simulink model "PRO_TestHarness"  (Simulink 8.6)
settings: Solver=ode45  StartTime=0.0  StopTime=10.0  RelTol=1e-3
PreLoadFcn:
  | addpath('./Workspace/')
  | load('./Workspace/EnvVar.mat')
  | if exist('tl_preloadfcn','file'), tl_preloadfcn(gcs,402); end
PostLoadFcn:
  | if exist('tl_postloadfcn','file'), tl_postloadfcn(gcs,402); end
InitFcn:
  | if exist('tlds_init','file'), tlds_init(gcs); end
StartFcn:
  | if exist('tlds_start','file'), tlds_start(gcs); end
StopFcn:
  | if exist('tlds_stop','file'), tlds_stop(gcs); end
undefined symbols (not defined in the file or in its folder): ddv, sigbuilder_block, Ts
libraries: tllib x19, simulink x2
(part 3 of 5)

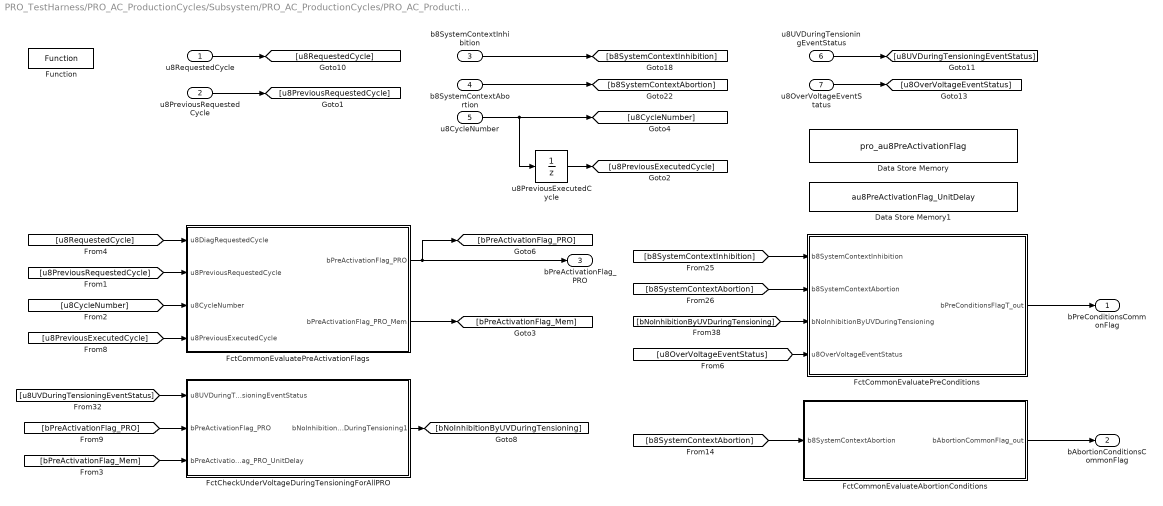
== system PRO_TestHarness/PRO_AC_ProductionCycles/Subsystem/PRO_AC_ProductionCycles/PRO_AC_ProductionCycles/PRO_runProductionCycles/PRO enabled/FctCommonPROManageInputs ==
  u8RequestedCycle : Inport  OutDataTypeStr=uint8  PortDimensions=1
  u8PreviousRequestedCycle : Inport  Port=2  OutDataTypeStr=uint8  PortDimensions=1
  b8SystemContextInhibition : Inport  Port=3  OutDataTypeStr=uint8  PortDimensions=1
  b8SystemContextAbortion : Inport  Port=4  OutDataTypeStr=uint8  PortDimensions=1
  u8CycleNumber : Inport  Port=5  PortDimensions=1
  u8UVDuringTensioningEventStatus : Inport  Port=6  OutDataTypeStr=uint8  PortDimensions=1
  u8OverVoltageEventStatus : Inport  Port=7
  Data Store Memory : DataStoreMemory  DataStoreName=pro_au8PreActivationFlag  ReadBeforeWriteMsg=warning  WriteAfterWriteMsg=warning  WriteAfterReadMsg=warning  InitialValue=ddv('PRO/pro_au8PreActivationFlag')  mask(TL_DataStoreMemory){data={'output',{'variable','PRO/pro_au8PreActivationFlag'},'autosar',{'softwarecomponent','AUTOLIV/SoftwareComponents/PRO/PRO_AC_ProductionCycles'},'date',736811.32661307871}}
      settings: CopyFcn=if exist('tl_reset_reviewflag') == 2, tl_reset_reviewflag(gcbh); end  DeleteFcn=if exist('delete_tlblock','file')==2,delete_tlblock(gcbh);end  NameChangeFcn=if exist('rename_tlblock','file')==2,rename_tlblock(gcbh);end  OpenFcn=if exist('tl_open_blockdlg','file')==2,tl_open_blockdlg(gcbh);else,open_system(gcbh,'parameter');end
      mask Help: eval(['if exist(''tl_online_help'',''file'') == 2, tl_online_help(''Topic'',''TL_DataStoreMemory''),else, web([''jar:file:///'',matlabroot,''/help/toolbox/simulink/help.jar!/slref/' lower(get_param(gcbh,'Blocktype')) '.html''], ''-helpbrowser''),end'])
      mask Display: plot([-0.05, 1.05, NaN, -0.05, 1.05],[.01, .01, NaN, .99, .99])
  Data Store Memory1 : DataStoreMemory  DataStoreName=au8PreActivationFlag_UnitDelay  ReadBeforeWriteMsg=warning  WriteAfterWriteMsg=warning  WriteAfterReadMsg=warning  InitialValue=ddv('PRO/pro_au8PreActivationFlag_UnitDelay')  mask(TL_DataStoreMemory){data={'output',{'variable','PRO/pro_au8PreActivationFlag_UnitDelay'},'autosar',{'softwarecomponent','AUTOLIV/SoftwareComponents/PRO/PRO_AC_ProductionCycles'},'date',736811.32661339117}}
      settings: CopyFcn=if exist('tl_reset_reviewflag') == 2, tl_reset_reviewflag(gcbh); end  DeleteFcn=if exist('delete_tlblock','file')==2,delete_tlblock(gcbh);end  NameChangeFcn=if exist('rename_tlblock','file')==2,rename_tlblock(gcbh);end  OpenFcn=if exist('tl_open_blockdlg','file')==2,tl_open_blockdlg(gcbh);else,open_system(gcbh,'parameter');end
      mask Help: eval(['if exist(''tl_online_help'',''file'') == 2, tl_online_help(''Topic'',''TL_DataStoreMemory''),else, web([''jar:file:///'',matlabroot,''/help/toolbox/simulink/help.jar!/slref/' lower(get_param(gcbh,'Blocktype')) '.html''], ''-helpbrowser''),end'])
      mask Display: plot([-0.05, 1.05, NaN, -0.05, 1.05],[.01, .01, NaN, .99, .99])
  FctCheckUnderVoltageDuringTensioningForAllPRO : Subsystem  TreatAsAtomicUnit=on
  FctCommonEvaluateAbortionConditions : Subsystem  TreatAsAtomicUnit=on
  FctCommonEvaluatePreActivationFlags : Subsystem  TreatAsAtomicUnit=on
  FctCommonEvaluatePreConditions : Subsystem  TreatAsAtomicUnit=on
  Function : tllib/Function  data={'stepfunctionname','ManageCommonInputsForAllPRO','stepfunctionclass','STATIC_FCN_ASR4','codecomment',['This function is in charge of' char(10) 'providing the following outputs:' char(10) '' char(10) '- the common PRO preconditions flag' char(10) '- the common PRO abortion flag' char(10) '- the consistent cycle number requested by diagnostic' char(10) '' char(10) 'according to the inputs:' char(10) '' char(10) '- the cycle requested by diagnostic' char(10) '- the complement of the cycle requested by diagnostic' char(10) '- inhibition context' char(10) '- abortion context'],'module','PRO_AC_ProductionCycles','date',736463.55388090282}  displayString=FUNCTION
  u8PreviousExecutedCycle : UnitDelay  InitialCondition=ddv('RTE_DEFINES/KU8_NO_CYCLE')  SampleTime=-1  mask(TL_UnitDelay){data={'output',{'name','$B','type','UInt8'},'state',{'name','X_$B','type','UInt8'},'date',736811.34423484956}}
      settings: CopyFcn=if exist('tl_reset_reviewflag') == 2, tl_reset_reviewflag(gcbh); end  DeleteFcn=if exist('delete_tlblock','file')==2,delete_tlblock(gcbh);end  NameChangeFcn=if exist('rename_tlblock','file')==2,rename_tlblock(gcbh);end  OpenFcn=if exist('tl_open_blockdlg','file')==2,tl_open_blockdlg(gcbh);else,open_system(gcbh,'parameter');end
      mask Help: eval(['if exist(''tl_online_help'',''file'') == 2, tl_online_help(''Topic'',''TL_UnitDelay''),else, web([''jar:file:///'',matlabroot,''/help/toolbox/simulink/help.jar!/slref/' lower(get_param(gcbh,'Blocktype')) '.html''], ''-helpbrowser''),end'])
      mask Display: plot([-0.05, 1.05, NaN, -0.05, 1.05],[.01, .01, NaN, .99, .99])
  bPreConditionsCommonFlag : Outport  InitialOutput=[0]
  bAbortionConditionsCommonFlag : Outport  Port=2  InitialOutput=[0]
  bPreActivationFlag_PRO : Outport  Port=3  InitialOutput=[0]
  wires:
  u8RequestedCycle/1 -> [u8RequestedCycle]
  FctCommonEvaluatePreConditions/1(bPreConditionsFlagT_out) -> bPreConditionsCommonFlag/1
  FctCommonEvaluateAbortionConditions/1(bAbortionCommonFlag_out) -> bAbortionConditionsCommonFlag/1
  b8SystemContextInhibition/1 -> [b8SystemContextInhibition]
  b8SystemContextAbortion/1 -> [b8SystemContextAbortion]
  [b8SystemContextAbortion] -> FctCommonEvaluatePreConditions/2(b8SystemContextAbortion)
  [b8SystemContextInhibition] -> FctCommonEvaluatePreConditions/1(b8SystemContextInhibition)
  [b8SystemContextAbortion] -> FctCommonEvaluateAbortionConditions/1(b8SystemContextAbortion)
  FctCommonEvaluatePreActivationFlags/1(bPreActivationFlag_PRO) -> [bPreActivationFlag_PRO], bPreActivationFlag_PRO/1
  [u8RequestedCycle] -> FctCommonEvaluatePreActivationFlags/1(u8DiagRequestedCycle)
  [u8PreviousRequestedCycle] -> FctCommonEvaluatePreActivationFlags/2(u8PreviousRequestedCycle)
  [u8CycleNumber] -> FctCommonEvaluatePreActivationFlags/3(u8CycleNumber)
  [u8PreviousExecutedCycle] -> FctCommonEvaluatePreActivationFlags/4(u8PreviousExecutedCycle)
  u8CycleNumber/1 -> u8PreviousExecutedCycle/1, [u8CycleNumber]
  u8PreviousExecutedCycle/1 -> [u8PreviousExecutedCycle]
  u8UVDuringTensioningEventStatus/1 -> [u8UVDuringTensioningEventStatus]
  FctCheckUnderVoltageDuringTensioningForAllPRO/1(bNoInhibitionByUVDuringTensioning1) -> [bNoInhibitionByUVDuringTensioning]
  [u8UVDuringTensioningEventStatus] -> FctCheckUnderVoltageDuringTensioningForAllPRO/1(u8UVDuringTensioningEventStatus)
  [bPreActivationFlag_PRO] -> FctCheckUnderVoltageDuringTensioningForAllPRO/2(bPreActivationFlag_PRO)
  [bNoInhibitionByUVDuringTensioning] -> FctCommonEvaluatePreConditions/3(bNoInhibitionByUVDuringTensioning)
  [u8OverVoltageEventStatus] -> FctCommonEvaluatePreConditions/4(u8OverVoltageEventStatus)
  u8OverVoltageEventStatus/1 -> [u8OverVoltageEventStatus]
  u8PreviousRequestedCycle/1 -> [u8PreviousRequestedCycle]
  [bPreActivationFlag_Mem] -> FctCheckUnderVoltageDuringTensioningForAllPRO/3(bPreActivationFlag_PRO_UnitDelay)
  FctCommonEvaluatePreActivationFlags/2(bPreActivationFlag_PRO_Mem) -> [bPreActivationFlag_Mem]

== system PRO_TestHarness/PRO_AC_ProductionCycles/Subsystem/PRO_AC_ProductionCycles/PRO_AC_ProductionCycles/PRO_runProductionCycles/PRO enabled/FctTrigAbortCycle_AllPRO ==
  u8ConsistentRequestedCycle : Inport  OutDataTypeStr=uint8  PortDimensions=1
  u8PreviousConsistentRequestedCycle1 : Inport  Port=2  OutDataTypeStr=uint8  PortDimensions=1
  u8ExecutedCycle : Inport  Port=3  PortDimensions=1
  bPreConditionsCommonFlag : Inport  Port=4
  bAbortionCommonFlag : Inport  Port=5  PortDimensions=1
  bPreActivation_PRO : Inport  Port=6
  Constant : Constant  Value=ddv('PRO/KU8_NB_PROD_CYCLE')  mask(TL_Constant){data={'output',{'variable','PRO/KU8_NB_PROD_CYCLE'},'date',736169.6247268056}}
      settings: CopyFcn=if exist('tl_reset_reviewflag') == 2, tl_reset_reviewflag(gcbh); end  DeleteFcn=if exist('delete_tlblock','file')==2,delete_tlblock(gcbh);end  NameChangeFcn=if exist('rename_tlblock','file')==2,rename_tlblock(gcbh);end  OpenFcn=if exist('tl_open_blockdlg','file')==2,tl_open_blockdlg(gcbh);else,open_system(gcbh,'parameter');end
      mask Help: eval(['if exist(''tl_online_help'',''file'') == 2, tl_online_help(''Topic'',''TL_Constant''),else, web([''jar:file:///'',matlabroot,''/help/toolbox/simulink/help.jar!/slref/' lower(get_param(gcbh,'Blocktype')) '.html''], ''-helpbrowser''),end'])
      mask Display: plot([-0.05, 1.05, NaN, -0.05, 1.05],[.01, .01, NaN, .99, .99])
  For Iterator Subsystem : Subsystem  TreatAsAtomicUnit=on
  Function : tllib/Function  data={'stepfunctionname','DecideForAllPRO','stepfunctionclass','STATIC_FCN_ASR4','codecomment',['This function is in charge of' char(10) 'providing the following outputs:' char(10) '' char(10) '- Trigger flags for PRO1 and PRO2 cycles' char(10) '- Pre Activation flags for PRO1 and PRO2 cycles' char(10) '- Pre Conditions flags for PRO1 and PRO2 cycles' char(10) '- Triggering Sources for PRO1 and PRO2 cycles' char(10) '' char(10) 'according to the inputs:' char(10) '' char(10) '- executed cycle number' char(10) '- consistent current cycle requested by diagnostic' char(10) '- common PRO preconditions flag' char(10) '- common PRO abortion flag'],'module','PRO_AC_ProductionCycles','date',736463.55393209495}  displayString=FUNCTION
  s8TempIndex : DataTypeConversion  mask(TL_Rescaler){data={'output',{'name','$B','type','Int8'},'date',736169.64125245367}}
      settings: DeleteFcn=if exist('delete_tlblock','file')==2,delete_tlblock(gcbh);end  NameChangeFcn=if exist('rename_tlblock','file')==2,rename_tlblock(gcbh);end  OpenFcn=if exist('tl_open_blockdlg','file')==2,tl_open_blockdlg(gcbh);else,open_system(gcbh,'parameter');end
      mask Help: eval(['if exist(''tl_online_help'',''file'') == 2, tl_online_help(''Topic'',''TL_Rescaler''),else, web([''jar:file:///'',matlabroot,''/help/toolbox/simulink/help.jar!/slref/' lower(get_param(gcbh,'Blocktype')) '.html''], ''-helpbrowser''),end'])
      mask Display: plot([-0.05, 1.05, NaN, -0.05, 1.05],[.01, .01, NaN, .99, .99])
  psrAlgoFlags_PRO1 : Outport
  psrAlgoFlags_PRO2 : Outport  Port=2
  wires:
  u8ExecutedCycle/1 -> [u8ExecutedCycle]
  bAbortionCommonFlag/1 -> [bAbortionCommonFlag]
  bPreConditionsCommonFlag/1 -> [bPreConditionsCommonFlag]
  u8ConsistentRequestedCycle/1 -> [u8RequestedCycle]
  bPreActivation_PRO/1 -> [bPreActivation_PRO]
  u8PreviousConsistentRequestedCycle1/1 -> [u8PreviousRequestedCycle]
  Constant/1 -> s8TempIndex/1
  s8TempIndex/1 -> For Iterator Subsystem/1(Iteration Limit)
  [bPreConditionsCommonFlag] -> For Iterator Subsystem/5(bPreConditionsCommonFlag)
  [bPreActivation_PRO] -> For Iterator Subsystem/7(bPreActivation_PRO)
  [bAbortionCommonFlag] -> For Iterator Subsystem/6(bAbortionCommonFlag)
  [u8PreviousRequestedCycle] -> For Iterator Subsystem/3(u8PreviousConsistentRequestedCycle1)
  [u8RequestedCycle] -> For Iterator Subsystem/2(u8ConsistentRequestedCycle)
  [u8ExecutedCycle] -> For Iterator Subsystem/4(u8ExecutedCycle)
  For Iterator Subsystem/1(psrAlgoFlags_PRO1) -> psrAlgoFlags_PRO1/1
  For Iterator Subsystem/2(psrAlgoFlags_PRO2) -> psrAlgoFlags_PRO2/1

== system PRO_TestHarness/PRO_AC_ProductionCycles/Subsystem/PRO_AC_ProductionCycles/PRO_AC_ProductionCycles/PRO_runProductionCycles/SCA_runCheckSystemContext1/If Action Subsystem1 ==
  Action Port : ActionPort  ActionType=then
  Data Store Read1 : DataStoreRead  DataStoreName=b8CyclesInhibitedByDTC  mask(TL_DataStoreRead){data={'date',735893.56911439809}}
      settings: DeleteFcn=if exist('delete_tlblock','file')==2,delete_tlblock(gcbh);end  NameChangeFcn=if exist('rename_tlblock','file')==2,rename_tlblock(gcbh);end  OpenFcn=if exist('tl_open_blockdlg','file')==2,tl_open_blockdlg(gcbh);else,open_system(gcbh,'parameter');end
      mask Help: eval(['if exist(''tl_online_help'',''file'') == 2, tl_online_help(''Topic'',''TL_DataStoreRead''),else, web([''jar:file:///'',matlabroot,''/help/toolbox/simulink/help.jar!/slref/' lower(get_param(gcbh,'Blocktype')) '.html''], ''-helpbrowser''),end'])
      mask Display: plot([-0.05, 1.05, NaN, -0.05, 1.05],[.01, .01, NaN, .99, .99])
  Out1 : Outport
  wires:
  Data Store Read1/1 -> Out1/1

== system PRO_TestHarness/PRO_AC_ProductionCycles/Subsystem/PRO_AC_ProductionCycles/PRO_AC_ProductionCycles/PRO_runProductionCycles/SCA_runCheckSystemContext1/If Action Subsystem2 ==
  Action Port : ActionPort  ActionType=else
  Data Store Read2 : DataStoreRead  DataStoreName=b8CyclesAbortedByDTC  mask(TL_DataStoreRead){data={'date',735893.56919435191}}
      settings: DeleteFcn=if exist('delete_tlblock','file')==2,delete_tlblock(gcbh);end  NameChangeFcn=if exist('rename_tlblock','file')==2,rename_tlblock(gcbh);end  OpenFcn=if exist('tl_open_blockdlg','file')==2,tl_open_blockdlg(gcbh);else,open_system(gcbh,'parameter');end
      mask Help: eval(['if exist(''tl_online_help'',''file'') == 2, tl_online_help(''Topic'',''TL_DataStoreRead''),else, web([''jar:file:///'',matlabroot,''/help/toolbox/simulink/help.jar!/slref/' lower(get_param(gcbh,'Blocktype')) '.html''], ''-helpbrowser''),end'])
      mask Display: plot([-0.05, 1.05, NaN, -0.05, 1.05],[.01, .01, NaN, .99, .99])
  Out1 : Outport
  wires:
  Data Store Read2/1 -> Out1/1

== system PRO_TestHarness/PRO_AC_ProductionCycles/Subsystem/PRO_AC_ProductionCycles/PRO_AC_ProductionCycles/PRO_runProductionCycles/SCA_runCheckSystemContext2/If Action Subsystem1 ==
  Action Port : ActionPort  ActionType=then
  Data Store Read1 : DataStoreRead  DataStoreName=b8CyclesInhibitedByDTC  mask(TL_DataStoreRead){data={'date',735893.5693029745}}
      settings: DeleteFcn=if exist('delete_tlblock','file')==2,delete_tlblock(gcbh);end  NameChangeFcn=if exist('rename_tlblock','file')==2,rename_tlblock(gcbh);end  OpenFcn=if exist('tl_open_blockdlg','file')==2,tl_open_blockdlg(gcbh);else,open_system(gcbh,'parameter');end
      mask Help: eval(['if exist(''tl_online_help'',''file'') == 2, tl_online_help(''Topic'',''TL_DataStoreRead''),else, web([''jar:file:///'',matlabroot,''/help/toolbox/simulink/help.jar!/slref/' lower(get_param(gcbh,'Blocktype')) '.html''], ''-helpbrowser''),end'])
      mask Display: plot([-0.05, 1.05, NaN, -0.05, 1.05],[.01, .01, NaN, .99, .99])
  Out1 : Outport
  wires:
  Data Store Read1/1 -> Out1/1

== system PRO_TestHarness/PRO_AC_ProductionCycles/Subsystem/PRO_AC_ProductionCycles/PRO_AC_ProductionCycles/PRO_runProductionCycles/SCA_runCheckSystemContext2/If Action Subsystem2 ==
  Action Port : ActionPort  ActionType=else
  Data Store Read2 : DataStoreRead  DataStoreName=b8CyclesAbortedByDTC  mask(TL_DataStoreRead){data={'date',735893.56938277779}}
      settings: DeleteFcn=if exist('delete_tlblock','file')==2,delete_tlblock(gcbh);end  NameChangeFcn=if exist('rename_tlblock','file')==2,rename_tlblock(gcbh);end  OpenFcn=if exist('tl_open_blockdlg','file')==2,tl_open_blockdlg(gcbh);else,open_system(gcbh,'parameter');end
      mask Help: eval(['if exist(''tl_online_help'',''file'') == 2, tl_online_help(''Topic'',''TL_DataStoreRead''),else, web([''jar:file:///'',matlabroot,''/help/toolbox/simulink/help.jar!/slref/' lower(get_param(gcbh,'Blocktype')) '.html''], ''-helpbrowser''),end'])
      mask Display: plot([-0.05, 1.05, NaN, -0.05, 1.05],[.01, .01, NaN, .99, .99])
  Out1 : Outport
  wires:
  Data Store Read2/1 -> Out1/1

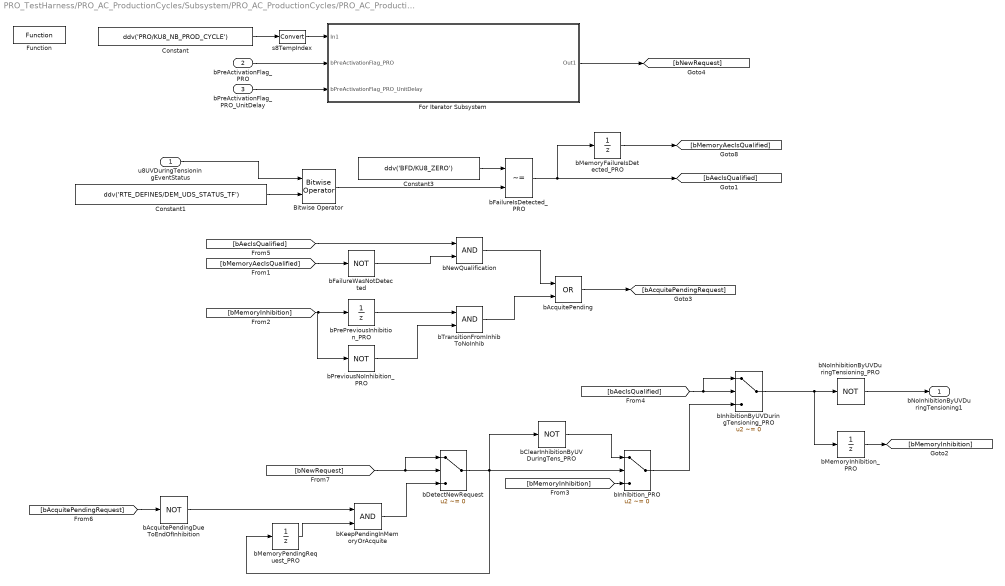
== system PRO_TestHarness/PRO_AC_ProductionCycles/Subsystem/PRO_AC_ProductionCycles/PRO_AC_ProductionCycles/PRO_runProductionCycles/PRO enabled/FctCommonPROManageInputs/FctCheckUnderVoltageDuringTensioningForAllPRO ==
  u8UVDuringTensioningEventStatus : Inport  OutDataTypeStr=uint8  PortDimensions=1
  bPreActivationFlag_PRO : Inport  Port=2
  bPreActivationFlag_PRO_UnitDelay : Inport  Port=3
  Bitwise Operator : tllib/Bitwise Operator  logicop=AND  UseBitMask=off  NumInputPorts=2  BitMask=bin2dec('11011001')  BitMaskRealWorld=Stored Integer  data={'date',736229.48596016201}
  Constant : Constant  Value=ddv('PRO/KU8_NB_PROD_CYCLE')  mask(TL_Constant){data={'output',{'variable','PRO/KU8_NB_PROD_CYCLE'},'date',736169.6247268056}}
      settings: CopyFcn=if exist('tl_reset_reviewflag') == 2, tl_reset_reviewflag(gcbh); end  DeleteFcn=if exist('delete_tlblock','file')==2,delete_tlblock(gcbh);end  NameChangeFcn=if exist('rename_tlblock','file')==2,rename_tlblock(gcbh);end  OpenFcn=if exist('tl_open_blockdlg','file')==2,tl_open_blockdlg(gcbh);else,open_system(gcbh,'parameter');end
      mask Help: eval(['if exist(''tl_online_help'',''file'') == 2, tl_online_help(''Topic'',''TL_Constant''),else, web([''jar:file:///'',matlabroot,''/help/toolbox/simulink/help.jar!/slref/' lower(get_param(gcbh,'Blocktype')) '.html''], ''-helpbrowser''),end'])
      mask Display: plot([-0.05, 1.05, NaN, -0.05, 1.05],[.01, .01, NaN, .99, .99])
  Constant1 : Constant  Value=ddv('RTE_DEFINES/DEM_UDS_STATUS_TF')  OutDataTypeStr=uint8  mask(TL_Constant){data={'output',{'variable','RTE_DEFINES/DEM_UDS_STATUS_TF'},'date',736811.33641298616}}
      settings: DeleteFcn=if exist('delete_tlblock','file')==2,delete_tlblock(gcbh);end  NameChangeFcn=if exist('rename_tlblock','file')==2,rename_tlblock(gcbh);end  OpenFcn=if exist('tl_open_blockdlg','file')==2,tl_open_blockdlg(gcbh);else,open_system(gcbh,'parameter');end
      mask Help: eval(['if exist(''tl_online_help'',''file'') == 2, tl_online_help(''Topic'',''TL_Constant''),else, web([''jar:file:///'',matlabroot,''/help/toolbox/simulink/help.jar!/slref/' lower(get_param(gcbh,'Blocktype')) '.html''], ''-helpbrowser''),end'])
      mask Display: plot([-0.05, 1.05, NaN, -0.05, 1.05],[.01, .01, NaN, .99, .99])
  Constant3 : Constant  Value=ddv('BFD/KU8_ZERO')  OutDataTypeStr=uint8  mask(TL_Constant){data={'output',{'variable','BFD/KU8_ZERO'},'date',736229.48516401625}}
      settings: DeleteFcn=if exist('delete_tlblock','file')==2,delete_tlblock(gcbh);end  NameChangeFcn=if exist('rename_tlblock','file')==2,rename_tlblock(gcbh);end  OpenFcn=if exist('tl_open_blockdlg','file')==2,tl_open_blockdlg(gcbh);else,open_system(gcbh,'parameter');end
      mask Help: eval(['if exist(''tl_online_help'',''file'') == 2, tl_online_help(''Topic'',''TL_Constant''),else, web([''jar:file:///'',matlabroot,''/help/toolbox/simulink/help.jar!/slref/' lower(get_param(gcbh,'Blocktype')) '.html''], ''-helpbrowser''),end'])
      mask Display: plot([-0.05, 1.05, NaN, -0.05, 1.05],[.01, .01, NaN, .99, .99])
  For Iterator Subsystem : Subsystem  TreatAsAtomicUnit=on
  Function : tllib/Function  data={'stepfunctionname','ExecuteBP_CheckUnderVoltageDuringTensioningForAllPRO','stepfunctionclass','STATIC_FCN_ASR4','codecomment',['This function is in charge of' char(10) 'providing the following outputs:' char(10) '' char(10) '- detection of temperature in correct range' char(10) '' char(10) 'according to the inputs:' char(10) '' char(10) '- the filtered internal temperature'],'module','PRO_AC_ProductionCycles','date',736463.55388949078}  displayString=FUNCTION
  bAcquitePending : Logic  Operator=OR  AllPortsSameDT=off  OutDataTypeStr=boolean  mask(TL_LogicalOperator){data={'output',{'name','$B'},'date',735916.64078504627}}
      settings: DeleteFcn=if exist('delete_tlblock','file')==2,delete_tlblock(gcbh);end  NameChangeFcn=if exist('rename_tlblock','file')==2,rename_tlblock(gcbh);end  OpenFcn=if exist('tl_open_blockdlg','file')==2,tl_open_blockdlg(gcbh);else,open_system(gcbh,'parameter');end
      mask Help: eval(['if exist(''tl_online_help'',''file'') == 2, tl_online_help(''Topic'',''TL_LogicalOperator''),else, web([''jar:file:///'',matlabroot,''/help/toolbox/simulink/help.jar!/slref/' lower(get_param(gcbh,'Blocktype')) '.html''], ''-helpbrowser''),end'])
      mask Display: plot([-0.05, 1.05, NaN, -0.05, 1.05],[.01, .01, NaN, .99, .99])
  bAcquitePendingDueToEndOfInhibition : Logic  Operator=NOT  Inputs=1  AllPortsSameDT=off  OutDataTypeStr=boolean  mask(TL_LogicalOperator){data={'output',{'name','$B'},'date',735910.63061995374}}
      settings: DeleteFcn=if exist('delete_tlblock','file')==2,delete_tlblock(gcbh);end  NameChangeFcn=if exist('rename_tlblock','file')==2,rename_tlblock(gcbh);end  OpenFcn=if exist('tl_open_blockdlg','file')==2,tl_open_blockdlg(gcbh);else,open_system(gcbh,'parameter');end
      mask Help: eval(['if exist(''tl_online_help'',''file'') == 2, tl_online_help(''Topic'',''TL_LogicalOperator''),else, web([''jar:file:///'',matlabroot,''/help/toolbox/simulink/help.jar!/slref/' lower(get_param(gcbh,'Blocktype')) '.html''], ''-helpbrowser''),end'])
      mask Display: plot([-0.05, 1.05, NaN, -0.05, 1.05],[.01, .01, NaN, .99, .99])
  bClearInhibitionByUVDuringTens_PRO : Logic  Operator=NOT  Inputs=1  AllPortsSameDT=off  OutDataTypeStr=boolean  mask(TL_LogicalOperator){data={'output',{'name','$B'},'date',735910.63061995374}}
      settings: DeleteFcn=if exist('delete_tlblock','file')==2,delete_tlblock(gcbh);end  NameChangeFcn=if exist('rename_tlblock','file')==2,rename_tlblock(gcbh);end  OpenFcn=if exist('tl_open_blockdlg','file')==2,tl_open_blockdlg(gcbh);else,open_system(gcbh,'parameter');end
      mask Help: eval(['if exist(''tl_online_help'',''file'') == 2, tl_online_help(''Topic'',''TL_LogicalOperator''),else, web([''jar:file:///'',matlabroot,''/help/toolbox/simulink/help.jar!/slref/' lower(get_param(gcbh,'Blocktype')) '.html''], ''-helpbrowser''),end'])
      mask Display: plot([-0.05, 1.05, NaN, -0.05, 1.05],[.01, .01, NaN, .99, .99])
  bDetectNewRequest : Switch  Criteria=u2 ~= 0  mask(TL_Switch){data={'output',{'name','$B','type','Bool'},'date',735907.68205655087}}
      settings: CopyFcn=if exist('tl_reset_reviewflag') == 2, tl_reset_reviewflag(gcbh); end  DeleteFcn=if exist('delete_tlblock','file')==2,delete_tlblock(gcbh);end  NameChangeFcn=if exist('rename_tlblock','file')==2,rename_tlblock(gcbh);end  OpenFcn=if exist('tl_open_blockdlg','file')==2,tl_open_blockdlg(gcbh);else,open_system(gcbh,'parameter');end
      mask Help: eval(['if exist(''tl_online_help'',''file'') == 2, tl_online_help(''Topic'',''TL_Switch''),else, web([''jar:file:///'',matlabroot,''/help/toolbox/simulink/help.jar!/slref/' lower(get_param(gcbh,'Blocktype')) '.html''], ''-helpbrowser''),end'])
      mask Display: plot([-0.05, 1.05, NaN, -0.05, 1.05],[.01, .01, NaN, .99, .99])
  bFailureIsDetected_PRO : RelationalOperator  Operator=~=  OutDataTypeStr=boolean  mask(TL_RelationalOperator){data={'output',{'name','$B'},'date',736229.48553751153}}
      settings: DeleteFcn=if exist('delete_tlblock','file')==2,delete_tlblock(gcbh);end  NameChangeFcn=if exist('rename_tlblock','file')==2,rename_tlblock(gcbh);end  OpenFcn=if exist('tl_open_blockdlg','file')==2,tl_open_blockdlg(gcbh);else,open_system(gcbh,'parameter');end
      mask Help: eval(['if exist(''tl_online_help'',''file'') == 2, tl_online_help(''Topic'',''TL_RelationalOperator''),else, web([''jar:file:///'',matlabroot,''/help/toolbox/simulink/help.jar!/slref/' lower(get_param(gcbh,'Blocktype')) '.html''], ''-helpbrowser''),end'])
      mask Display: plot([-0.05, 1.05, NaN, -0.05, 1.05],[.01, .01, NaN, .99, .99])
  bFailureWasNotDetected : Logic  Operator=NOT  Inputs=1  AllPortsSameDT=off  OutDataTypeStr=boolean  mask(TL_LogicalOperator){data={'output',{'name','$B'},'date',735910.63061995374}}
      settings: DeleteFcn=if exist('delete_tlblock','file')==2,delete_tlblock(gcbh);end  NameChangeFcn=if exist('rename_tlblock','file')==2,rename_tlblock(gcbh);end  OpenFcn=if exist('tl_open_blockdlg','file')==2,tl_open_blockdlg(gcbh);else,open_system(gcbh,'parameter');end
      mask Help: eval(['if exist(''tl_online_help'',''file'') == 2, tl_online_help(''Topic'',''TL_LogicalOperator''),else, web([''jar:file:///'',matlabroot,''/help/toolbox/simulink/help.jar!/slref/' lower(get_param(gcbh,'Blocktype')) '.html''], ''-helpbrowser''),end'])
      mask Display: plot([-0.05, 1.05, NaN, -0.05, 1.05],[.01, .01, NaN, .99, .99])
  bInhibitionByUVDuringTensioning_PRO : Switch  Criteria=u2 ~= 0  mask(TL_Switch){data={'output',{'name','$B','type','Bool'},'date',735907.68205655087}}
      settings: CopyFcn=if exist('tl_reset_reviewflag') == 2, tl_reset_reviewflag(gcbh); end  DeleteFcn=if exist('delete_tlblock','file')==2,delete_tlblock(gcbh);end  NameChangeFcn=if exist('rename_tlblock','file')==2,rename_tlblock(gcbh);end  OpenFcn=if exist('tl_open_blockdlg','file')==2,tl_open_blockdlg(gcbh);else,open_system(gcbh,'parameter');end
      mask Help: eval(['if exist(''tl_online_help'',''file'') == 2, tl_online_help(''Topic'',''TL_Switch''),else, web([''jar:file:///'',matlabroot,''/help/toolbox/simulink/help.jar!/slref/' lower(get_param(gcbh,'Blocktype')) '.html''], ''-helpbrowser''),end'])
      mask Display: plot([-0.05, 1.05, NaN, -0.05, 1.05],[.01, .01, NaN, .99, .99])
  bInhibition_PRO : Switch  Criteria=u2 ~= 0  mask(TL_Switch){data={'output',{'name','$B','type','Bool'},'date',735907.68205655087}}
      settings: CopyFcn=if exist('tl_reset_reviewflag') == 2, tl_reset_reviewflag(gcbh); end  DeleteFcn=if exist('delete_tlblock','file')==2,delete_tlblock(gcbh);end  NameChangeFcn=if exist('rename_tlblock','file')==2,rename_tlblock(gcbh);end  OpenFcn=if exist('tl_open_blockdlg','file')==2,tl_open_blockdlg(gcbh);else,open_system(gcbh,'parameter');end
      mask Help: eval(['if exist(''tl_online_help'',''file'') == 2, tl_online_help(''Topic'',''TL_Switch''),else, web([''jar:file:///'',matlabroot,''/help/toolbox/simulink/help.jar!/slref/' lower(get_param(gcbh,'Blocktype')) '.html''], ''-helpbrowser''),end'])
      mask Display: plot([-0.05, 1.05, NaN, -0.05, 1.05],[.01, .01, NaN, .99, .99])
  bKeepPendingInMemoryOrAcquite : Logic  AllPortsSameDT=off  OutDataTypeStr=boolean  mask(TL_LogicalOperator){data={'output',{'name','$B'},'date',735907.68610908568}}
      settings: DeleteFcn=if exist('delete_tlblock','file')==2,delete_tlblock(gcbh);end  NameChangeFcn=if exist('rename_tlblock','file')==2,rename_tlblock(gcbh);end  OpenFcn=if exist('tl_open_blockdlg','file')==2,tl_open_blockdlg(gcbh);else,open_system(gcbh,'parameter');end
      mask Help: eval(['if exist(''tl_online_help'',''file'') == 2, tl_online_help(''Topic'',''TL_LogicalOperator''),else, web([''jar:file:///'',matlabroot,''/help/toolbox/simulink/help.jar!/slref/' lower(get_param(gcbh,'Blocktype')) '.html''], ''-helpbrowser''),end'])
      mask Display: plot([-0.05, 1.05, NaN, -0.05, 1.05],[.01, .01, NaN, .99, .99])
  bMemoryFailureIsDetected_PRO : UnitDelay  SampleTime=-1  mask(TL_UnitDelay){data={'output',{'name','$B','type','Bool'},'state',{'name','X_$B','type','Bool'},'date',735916.45127987268}}
      settings: CopyFcn=if exist('tl_reset_reviewflag') == 2, tl_reset_reviewflag(gcbh); end  DeleteFcn=if exist('delete_tlblock','file')==2,delete_tlblock(gcbh);end  NameChangeFcn=if exist('rename_tlblock','file')==2,rename_tlblock(gcbh);end  OpenFcn=if exist('tl_open_blockdlg','file')==2,tl_open_blockdlg(gcbh);else,open_system(gcbh,'parameter');end
      mask Help: eval(['if exist(''tl_online_help'',''file'') == 2, tl_online_help(''Topic'',''TL_UnitDelay''),else, web([''jar:file:///'',matlabroot,''/help/toolbox/simulink/help.jar!/slref/' lower(get_param(gcbh,'Blocktype')) '.html''], ''-helpbrowser''),end'])
      mask Display: plot([-0.05, 1.05, NaN, -0.05, 1.05],[.01, .01, NaN, .99, .99])
  bMemoryInhibition_PRO : UnitDelay  SampleTime=-1  mask(TL_UnitDelay){data={'output',{'name','$B','type','Bool'},'state',{'name','X_$B','type','Bool'},'date',735916.45127987268}}
      settings: CopyFcn=if exist('tl_reset_reviewflag') == 2, tl_reset_reviewflag(gcbh); end  DeleteFcn=if exist('delete_tlblock','file')==2,delete_tlblock(gcbh);end  NameChangeFcn=if exist('rename_tlblock','file')==2,rename_tlblock(gcbh);end  OpenFcn=if exist('tl_open_blockdlg','file')==2,tl_open_blockdlg(gcbh);else,open_system(gcbh,'parameter');end
      mask Help: eval(['if exist(''tl_online_help'',''file'') == 2, tl_online_help(''Topic'',''TL_UnitDelay''),else, web([''jar:file:///'',matlabroot,''/help/toolbox/simulink/help.jar!/slref/' lower(get_param(gcbh,'Blocktype')) '.html''], ''-helpbrowser''),end'])
      mask Display: plot([-0.05, 1.05, NaN, -0.05, 1.05],[.01, .01, NaN, .99, .99])
  bMemoryPendingRequest_PRO : UnitDelay  SampleTime=-1  mask(TL_UnitDelay){data={'output',{'name','$B','type','Bool'},'state',{'name','X_$B','type','Bool'},'date',735916.62110291666}}
      settings: CopyFcn=if exist('tl_reset_reviewflag') == 2, tl_reset_reviewflag(gcbh); end  DeleteFcn=if exist('delete_tlblock','file')==2,delete_tlblock(gcbh);end  NameChangeFcn=if exist('rename_tlblock','file')==2,rename_tlblock(gcbh);end  OpenFcn=if exist('tl_open_blockdlg','file')==2,tl_open_blockdlg(gcbh);else,open_system(gcbh,'parameter');end
      mask Help: eval(['if exist(''tl_online_help'',''file'') == 2, tl_online_help(''Topic'',''TL_UnitDelay''),else, web([''jar:file:///'',matlabroot,''/help/toolbox/simulink/help.jar!/slref/' lower(get_param(gcbh,'Blocktype')) '.html''], ''-helpbrowser''),end'])
      mask Display: plot([-0.05, 1.05, NaN, -0.05, 1.05],[.01, .01, NaN, .99, .99])
  bNewQualification : Logic  AllPortsSameDT=off  OutDataTypeStr=boolean  mask(TL_LogicalOperator){data={'output',{'name','$B'},'date',735907.68610908568}}
      settings: DeleteFcn=if exist('delete_tlblock','file')==2,delete_tlblock(gcbh);end  NameChangeFcn=if exist('rename_tlblock','file')==2,rename_tlblock(gcbh);end  OpenFcn=if exist('tl_open_blockdlg','file')==2,tl_open_blockdlg(gcbh);else,open_system(gcbh,'parameter');end
      mask Help: eval(['if exist(''tl_online_help'',''file'') == 2, tl_online_help(''Topic'',''TL_LogicalOperator''),else, web([''jar:file:///'',matlabroot,''/help/toolbox/simulink/help.jar!/slref/' lower(get_param(gcbh,'Blocktype')) '.html''], ''-helpbrowser''),end'])
      mask Display: plot([-0.05, 1.05, NaN, -0.05, 1.05],[.01, .01, NaN, .99, .99])
  bNoInhibitionByUVDuringTensioning_PRO : Logic  Operator=NOT  Inputs=1  AllPortsSameDT=off  OutDataTypeStr=boolean  mask(TL_LogicalOperator){data={'output',{'name','$B'},'date',735916.41568038194}}
      settings: DeleteFcn=if exist('delete_tlblock','file')==2,delete_tlblock(gcbh);end  NameChangeFcn=if exist('rename_tlblock','file')==2,rename_tlblock(gcbh);end  OpenFcn=if exist('tl_open_blockdlg','file')==2,tl_open_blockdlg(gcbh);else,open_system(gcbh,'parameter');end
      mask Help: eval(['if exist(''tl_online_help'',''file'') == 2, tl_online_help(''Topic'',''TL_LogicalOperator''),else, web([''jar:file:///'',matlabroot,''/help/toolbox/simulink/help.jar!/slref/' lower(get_param(gcbh,'Blocktype')) '.html''], ''-helpbrowser''),end'])
      mask Display: plot([-0.05, 1.05, NaN, -0.05, 1.05],[.01, .01, NaN, .99, .99])
  bPrePreviousInhibition_PRO : UnitDelay  SampleTime=-1  mask(TL_UnitDelay){data={'output',{'name','$B','type','Bool'},'state',{'name','X_$B','type','Bool'},'date',735916.62723281246}}
      settings: CopyFcn=if exist('tl_reset_reviewflag') == 2, tl_reset_reviewflag(gcbh); end  DeleteFcn=if exist('delete_tlblock','file')==2,delete_tlblock(gcbh);end  NameChangeFcn=if exist('rename_tlblock','file')==2,rename_tlblock(gcbh);end  OpenFcn=if exist('tl_open_blockdlg','file')==2,tl_open_blockdlg(gcbh);else,open_system(gcbh,'parameter');end
      mask Help: eval(['if exist(''tl_online_help'',''file'') == 2, tl_online_help(''Topic'',''TL_UnitDelay''),else, web([''jar:file:///'',matlabroot,''/help/toolbox/simulink/help.jar!/slref/' lower(get_param(gcbh,'Blocktype')) '.html''], ''-helpbrowser''),end'])
      mask Display: plot([-0.05, 1.05, NaN, -0.05, 1.05],[.01, .01, NaN, .99, .99])
  bPreviousNoInhibition_PRO : Logic  Operator=NOT  Inputs=1  AllPortsSameDT=off  OutDataTypeStr=boolean  mask(TL_LogicalOperator){data={'output',{'name','$B'},'date',735910.63061995374}}
      settings: DeleteFcn=if exist('delete_tlblock','file')==2,delete_tlblock(gcbh);end  NameChangeFcn=if exist('rename_tlblock','file')==2,rename_tlblock(gcbh);end  OpenFcn=if exist('tl_open_blockdlg','file')==2,tl_open_blockdlg(gcbh);else,open_system(gcbh,'parameter');end
      mask Help: eval(['if exist(''tl_online_help'',''file'') == 2, tl_online_help(''Topic'',''TL_LogicalOperator''),else, web([''jar:file:///'',matlabroot,''/help/toolbox/simulink/help.jar!/slref/' lower(get_param(gcbh,'Blocktype')) '.html''], ''-helpbrowser''),end'])
      mask Display: plot([-0.05, 1.05, NaN, -0.05, 1.05],[.01, .01, NaN, .99, .99])
  bTransitionFromInhibToNoInhib : Logic  AllPortsSameDT=off  OutDataTypeStr=boolean  mask(TL_LogicalOperator){data={'output',{'name','$B'},'date',735907.68610908568}}
      settings: DeleteFcn=if exist('delete_tlblock','file')==2,delete_tlblock(gcbh);end  NameChangeFcn=if exist('rename_tlblock','file')==2,rename_tlblock(gcbh);end  OpenFcn=if exist('tl_open_blockdlg','file')==2,tl_open_blockdlg(gcbh);else,open_system(gcbh,'parameter');end
      mask Help: eval(['if exist(''tl_online_help'',''file'') == 2, tl_online_help(''Topic'',''TL_LogicalOperator''),else, web([''jar:file:///'',matlabroot,''/help/toolbox/simulink/help.jar!/slref/' lower(get_param(gcbh,'Blocktype')) '.html''], ''-helpbrowser''),end'])
      mask Display: plot([-0.05, 1.05, NaN, -0.05, 1.05],[.01, .01, NaN, .99, .99])
  s8TempIndex : DataTypeConversion  mask(TL_Rescaler){data={'output',{'name','$B','type','Int8'},'date',736169.64125245367}}
      settings: DeleteFcn=if exist('delete_tlblock','file')==2,delete_tlblock(gcbh);end  NameChangeFcn=if exist('rename_tlblock','file')==2,rename_tlblock(gcbh);end  OpenFcn=if exist('tl_open_blockdlg','file')==2,tl_open_blockdlg(gcbh);else,open_system(gcbh,'parameter');end
      mask Help: eval(['if exist(''tl_online_help'',''file'') == 2, tl_online_help(''Topic'',''TL_Rescaler''),else, web([''jar:file:///'',matlabroot,''/help/toolbox/simulink/help.jar!/slref/' lower(get_param(gcbh,'Blocktype')) '.html''], ''-helpbrowser''),end'])
      mask Display: plot([-0.05, 1.05, NaN, -0.05, 1.05],[.01, .01, NaN, .99, .99])
  bNoInhibitionByUVDuringTensioning1 : Outport  PortDimensions=1
  wires:
  bInhibitionByUVDuringTensioning_PRO/1 -> bMemoryInhibition_PRO/1, bNoInhibitionByUVDuringTensioning_PRO/1
  bNoInhibitionByUVDuringTensioning_PRO/1 -> bNoInhibitionByUVDuringTensioning1/1
  bDetectNewRequest/1 -> bMemoryPendingRequest_PRO/1, bInhibition_PRO/2, bClearInhibitionByUVDuringTens_PRO/1
  bInhibition_PRO/1 -> bInhibitionByUVDuringTensioning_PRO/3
  [bMemoryInhibition] -> bPreviousNoInhibition_PRO/1, bPrePreviousInhibition_PRO/1
  bPrePreviousInhibition_PRO/1 -> bTransitionFromInhibToNoInhib/1
  bPreviousNoInhibition_PRO/1 -> bTransitionFromInhibToNoInhib/2
  bClearInhibitionByUVDuringTens_PRO/1 -> bInhibition_PRO/1
  bKeepPendingInMemoryOrAcquite/1 -> bDetectNewRequest/3
  bMemoryPendingRequest_PRO/1 -> bKeepPendingInMemoryOrAcquite/2
  bMemoryFailureIsDetected_PRO/1 -> [bMemoryAecIsQualified]
  [bAecIsQualified] -> bNewQualification/1
  [bMemoryAecIsQualified] -> bFailureWasNotDetected/1
  bFailureWasNotDetected/1 -> bNewQualification/2
  bNewQualification/1 -> bAcquitePending/1
  bAcquitePendingDueToEndOfInhibition/1 -> bKeepPendingInMemoryOrAcquite/1
  bTransitionFromInhibToNoInhib/1 -> bAcquitePending/2
  bMemoryInhibition_PRO/1 -> [bMemoryInhibition]
  [bMemoryInhibition] -> bInhibition_PRO/3
  [bAecIsQualified] -> bInhibitionByUVDuringTensioning_PRO/1, bInhibitionByUVDuringTensioning_PRO/2
  bAcquitePending/1 -> [bAcquitePendingRequest]
  [bAcquitePendingRequest] -> bAcquitePendingDueToEndOfInhibition/1
  [bNewRequest] -> bDetectNewRequest/1, bDetectNewRequest/2
  Constant/1 -> s8TempIndex/1
  s8TempIndex/1 -> For Iterator Subsystem/1(In1)
  For Iterator Subsystem/1(Out1) -> [bNewRequest]
  bPreActivationFlag_PRO/1 -> For Iterator Subsystem/2(bPreActivationFlag_PRO)
  bPreActivationFlag_PRO_UnitDelay/1 -> For Iterator Subsystem/3(bPreActivationFlag_PRO_UnitDelay)
  Constant1/1 -> Bitwise Operator/2
  u8UVDuringTensioningEventStatus/1 -> Bitwise Operator/1
  Constant3/1 -> bFailureIsDetected_PRO/1
  Bitwise Operator/1 -> bFailureIsDetected_PRO/2
  bFailureIsDetected_PRO/1 -> bMemoryFailureIsDetected_PRO/1, [bAecIsQualified]

== system PRO_TestHarness/PRO_AC_ProductionCycles/Subsystem/PRO_AC_ProductionCycles/PRO_AC_ProductionCycles/PRO_runProductionCycles/PRO enabled/FctCommonPROManageInputs/FctCommonEvaluateAbortionConditions ==
  b8SystemContextAbortion : Inport  OutDataTypeStr=uint8  PortDimensions=1
  Constant4 : Constant  Value=ddv('BFD/KU8_CONTEXT_STATUS_ON')  OutDataTypeStr=uint8  mask(TL_Constant){data={'output',{'variable','BFD/KU8_CONTEXT_STATUS_ON'},'date',735893.58242832171}}
      settings: DeleteFcn=if exist('delete_tlblock','file')==2,delete_tlblock(gcbh);end  NameChangeFcn=if exist('rename_tlblock','file')==2,rename_tlblock(gcbh);end  OpenFcn=if exist('tl_open_blockdlg','file')==2,tl_open_blockdlg(gcbh);else,open_system(gcbh,'parameter');end
      mask Help: eval(['if exist(''tl_online_help'',''file'') == 2, tl_online_help(''Topic'',''TL_Constant''),else, web([''jar:file:///'',matlabroot,''/help/toolbox/simulink/help.jar!/slref/' lower(get_param(gcbh,'Blocktype')) '.html''], ''-helpbrowser''),end'])
      mask Display: plot([-0.05, 1.05, NaN, -0.05, 1.05],[.01, .01, NaN, .99, .99])
  Function : tllib/Function  data={'stepfunctionname','EvaluateAbortionConditionsForAllPRO','stepfunctionclass','STATIC_FCN_ASR4','codecomment',['This function is in charge of' char(10) 'providing the following outputs:' char(10) '' char(10) '- the common PRO abortion flag' char(10) '' char(10) 'according to the inputs:' char(10) '' char(10) '- abortion context'],'module','PRO_AC_ProductionCycles','date',736463.55390737264}  displayString=FUNCTION
  bAbortionCommonFlag_PRO : RelationalOperator  Operator===  OutDataTypeStr=boolean  mask(TL_RelationalOperator){data={'output',{'name','$B'},'date',735893.57217673608}}
      settings: DeleteFcn=if exist('delete_tlblock','file')==2,delete_tlblock(gcbh);end  NameChangeFcn=if exist('rename_tlblock','file')==2,rename_tlblock(gcbh);end  OpenFcn=if exist('tl_open_blockdlg','file')==2,tl_open_blockdlg(gcbh);else,open_system(gcbh,'parameter');end
      mask Help: eval(['if exist(''tl_online_help'',''file'') == 2, tl_online_help(''Topic'',''TL_RelationalOperator''),else, web([''jar:file:///'',matlabroot,''/help/toolbox/simulink/help.jar!/slref/' lower(get_param(gcbh,'Blocktype')) '.html''], ''-helpbrowser''),end'])
      mask Display: plot([-0.05, 1.05, NaN, -0.05, 1.05],[.01, .01, NaN, .99, .99])
  bAbortionCommonFlag_out : Outport  InitialOutput=[0]
  wires:
  bAbortionCommonFlag_PRO/1 -> bAbortionCommonFlag_out/1
  Constant4/1 -> bAbortionCommonFlag_PRO/2
  b8SystemContextAbortion/1 -> bAbortionCommonFlag_PRO/1

== system PRO_TestHarness/PRO_AC_ProductionCycles/Subsystem/PRO_AC_ProductionCycles/PRO_AC_ProductionCycles/PRO_runProductionCycles/PRO enabled/FctCommonPROManageInputs/FctCommonEvaluatePreActivationFlags ==
  u8DiagRequestedCycle : Inport  OutDataTypeStr=uint8  PortDimensions=1
  u8PreviousRequestedCycle : Inport  Port=2  OutDataTypeStr=uint8  PortDimensions=1
  u8CycleNumber : Inport  Port=3  PortDimensions=1
  u8PreviousExecutedCycle : Inport  Port=4  PortDimensions=1
  Constant : Constant  Value=ddv('PRO/KU8_NB_PROD_CYCLE')  mask(TL_Constant){data={'output',{'variable','PRO/KU8_NB_PROD_CYCLE'},'date',736169.6247268056}}
      settings: CopyFcn=if exist('tl_reset_reviewflag') == 2, tl_reset_reviewflag(gcbh); end  DeleteFcn=if exist('delete_tlblock','file')==2,delete_tlblock(gcbh);end  NameChangeFcn=if exist('rename_tlblock','file')==2,rename_tlblock(gcbh);end  OpenFcn=if exist('tl_open_blockdlg','file')==2,tl_open_blockdlg(gcbh);else,open_system(gcbh,'parameter');end
      mask Help: eval(['if exist(''tl_online_help'',''file'') == 2, tl_online_help(''Topic'',''TL_Constant''),else, web([''jar:file:///'',matlabroot,''/help/toolbox/simulink/help.jar!/slref/' lower(get_param(gcbh,'Blocktype')) '.html''], ''-helpbrowser''),end'])
      mask Display: plot([-0.05, 1.05, NaN, -0.05, 1.05],[.01, .01, NaN, .99, .99])
  For Iterator Subsystem : Subsystem  TreatAsAtomicUnit=on
  s8TempIndex : DataTypeConversion  mask(TL_Rescaler){data={'output',{'name','$B','type','Int8'},'date',736169.64125245367}}
      settings: DeleteFcn=if exist('delete_tlblock','file')==2,delete_tlblock(gcbh);end  NameChangeFcn=if exist('rename_tlblock','file')==2,rename_tlblock(gcbh);end  OpenFcn=if exist('tl_open_blockdlg','file')==2,tl_open_blockdlg(gcbh);else,open_system(gcbh,'parameter');end
      mask Help: eval(['if exist(''tl_online_help'',''file'') == 2, tl_online_help(''Topic'',''TL_Rescaler''),else, web([''jar:file:///'',matlabroot,''/help/toolbox/simulink/help.jar!/slref/' lower(get_param(gcbh,'Blocktype')) '.html''], ''-helpbrowser''),end'])
      mask Display: plot([-0.05, 1.05, NaN, -0.05, 1.05],[.01, .01, NaN, .99, .99])
  bPreActivationFlag_PRO : Outport  InitialOutput=[0]
  bPreActivationFlag_PRO_Mem : Outport  Port=2  InitialOutput=[0]
  wires:
  u8CycleNumber/1 -> [u8CycleNumber]
  u8DiagRequestedCycle/1 -> [u8RequestedCycle]
  u8PreviousExecutedCycle/1 -> [u8PreviousExecutedCycle]
  u8PreviousRequestedCycle/1 -> [u8PreviousRequestedCycle]
  Constant/1 -> s8TempIndex/1
  [u8RequestedCycle] -> For Iterator Subsystem/2(u8DiagRequestedCycle)
  [u8PreviousRequestedCycle] -> For Iterator Subsystem/3(u8PreviousRequestedCycle)
  [u8CycleNumber] -> For Iterator Subsystem/4(u8CycleNumber)
  [u8PreviousExecutedCycle] -> For Iterator Subsystem/5(u8PreviousExecutedCycle)
  s8TempIndex/1 -> For Iterator Subsystem/1(s8ProdCycleNb)
  For Iterator Subsystem/1(au8PreActivationFlag) -> bPreActivationFlag_PRO/1
  For Iterator Subsystem/2(au8PreActivationFlag_Mem) -> bPreActivationFlag_PRO_Mem/1
